simulink model "Back2BackSim1"  (R2017a)
settings: Solver=VariableStepAuto  StartTime=0.0  StopTime=.2  RelTol=1e-3
undefined symbols (not defined in the file or in its folder): st_time3
libraries: fl_lib x62, nesl_utility x32, powerlib_meascontrol x8, powerlib x1, elec_lib x1
(part 1 of 2)
settings Model: Creator=erich  LastModifiedBy=erich

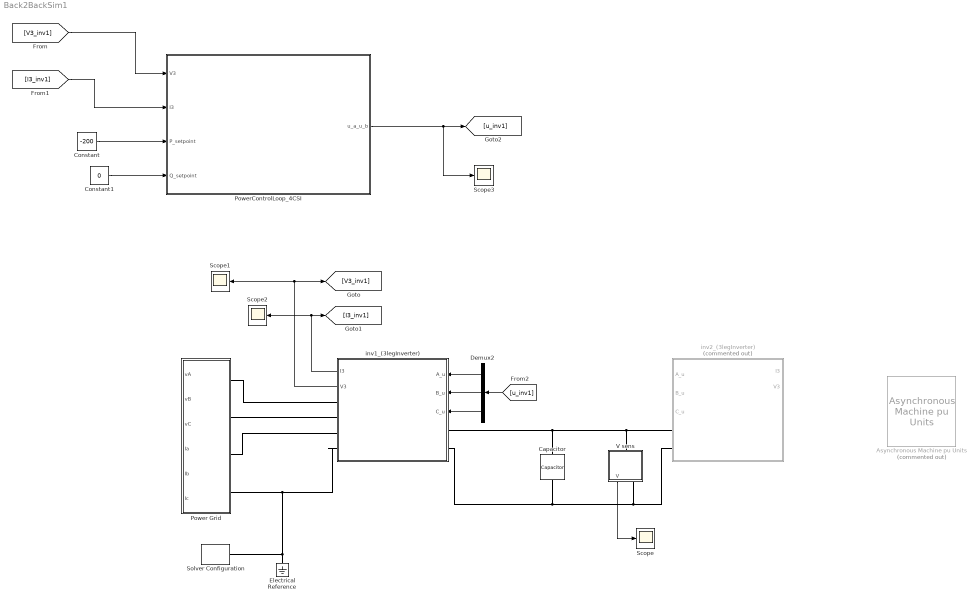
== system Back2BackSim1 ==
  Asynchronous Machine pu Units : powerlib/Machines/Asynchronous Machine pu Units  Commented=on  RotorType=Squirrel-cage  PresetModel=No  MechanicalLoad=Torque Tm  ShowDetailedParameters=on  ReferenceFrame=Rotor  Units=pu  MeasurementBus=off  NominalParameters=[3730 460 60]  Stator=[0.01965 0.0397]  Rotor=[0.01909 0.0397]  Cage1=[0.01909 0.0397]  Cage2=[0.01909 0.0397]  Lm=1.354  Mechanical=[0.09526 0.05479 2]  PolePairs=2  InitialConditions="[ 1,0   0,0,0   0,0,0 ]"  SimulateSaturation=off  Saturation="[0.212,0.4201,0.8125,1.0979,1.4799,2.2457,3.2586,4.5763,6.4763 ;   0.5,0.7,0.9,1,1.1,1.2 ,1.3,1.4,1.5]"  LoadFlowParameters=0  TsPowergui=0  TsBlock=-1  IterativeModel=Trapezoidal non iterative  IterativeDiscreteModel=Trapezoidal non iterative  Pmec=0
      settings: SourceProductName=Simscape Power Systems  SourceProductBaseCode=PS
  Capacitor : elec_lib/Passive Devices/Capacitor  enable_table=0  c=100 uF  Cvec=[1.0e-5, 1.0e-6] F  Vvec=[0.0, 10.0] V  CV_table_symmetry=1  C_tol=5  enable_C_tol=0  tol_distribution=1  nSigma=4  r=1e-6 Ohm  g=0 1/Ohm  enable_operating_limits=0  operating_limit_action=2  max_working_voltage_range=[-25.0, 25.0] V  power_rating=1 W  enable_faults=0  fault_action=1  Cscale_faulted=100  R_faulted=1e-3 Ohm  G_faulted=0 1/Ohm  tau_fault=1e-3 s  enable_temporal_fault=0  t_fault=1 s  enable_behavioral_fault=0  max_permissible_voltage_range=[-100.0, 100.0] V  t_fail_on_voltage=1 s  i_specify=off  i_priority=None  i=0 A  i_nominal_specify=off  i_nominal_unit=A  i_nominal_value=1  v_specify=off  v_priority=None  v=0 V  v_nominal_specify=off  v_nominal_unit=V  v_nominal_value=1  vc_specify=off  vc_priority=High  vc=0 V  vc_nominal_specify=off  vc_nominal_unit=V  vc_nominal_value=1
  Constant : Constant  Value=-200
  Constant1 : Constant  Value=0
  Demux2 : Demux  Outputs=3
  Electrical Reference : fl_lib/Electrical/Electrical Elements/Electrical Reference
  Power Grid : Subsystem
  PowerControlLoop_4CSI : Subsystem
      mask Display:
      | port_label('input', 1, '\fontsize{14} V_{abc}', 'texmode', 'on')
      | port_label('input', 2, '\fontsize{14} I_{abc}', 'texmode', 'on')
      | port_label('input', 3, '\fontsize{14} P_{set}', 'texmode', 'on')
      | port_label('input', 4, '\fontsize{14} Q_{set}', 'texmode', 'on')
      | port_label('output', 1, '\fontsize{14} u_{\alpha, \beta}', 'texmode', 'on')
      | 
      | 
      | disp('\fontsize{12} Power Control for 3\Phi CSI', 'texmode', 'on')
  Scope{,1..3} (4 alike) : Scope
  Solver Configuration : nesl_utility/Solver Configuration  PhysicalDomain=network_engine_domain  SubClassName=solver  LeftPortType=input  RightPortType=generic  Accelerate=off  Tones=[]  Harmonics=[]  SimulateNoise=off  Profile=off  UseLocalSampling=off  EnableSwitchedLinearOptims=on  FrequencyDomain=off  UseCCode=off  RelTol=0.001  AbsTol=1e-06  MinStep=1e-09  ToWorkspace=off  RevertToSquareIcSolve=off  NumHomotopyIterations=100  PhasorMode=off  PhasorModeNumHarmonics=1  OverrideAbsTol=off  DoDC=off  ResidualTolerance=1e-09  UseLocalSolver=on  LocalSolverChoice=NE_BACKWARD_EULER_ADVANCER  LocalSolverSampleTime=1e-6  DoFixedCost=on  MaxNonlinIter=3  MaxModeIter=2  LinearAlgebra=Sparse  DelaysMemoryBudget=1024  AutomaticFiltering=on  FilteringTimeConstant=0.001
  V sens : Subsystem
      mask Display:
      | port_label('lconn', 1, '+')
      | port_label('rconn', 1, '-')
      | port_label('output', 1, 'V')
      | 
      | 
      | x=.5+[-.31:.01:.31];
      | y=sqrt(.1-(x-.5).^2)+.4;
      | y2=-sqrt(.1-(x-.5).^2)+.5;
      | 
      | plot(x, y)
      | plot(x, y2)
      | 
      | text(.47, .5,'V', 'texmode', 'on')
      | 
      | plot([.1 .22], [.44 .44])
      | plot([.8 .9], [.44 .44])
  inv1_(3legInverter) : Subsystem
      mask Display:
      | port_label('input', 1, 'A_u')
      | port_label('input', 2, 'B_u')
      | port_label('input', 3, 'C_u')
      | 
      | port_label('lconn', 1, 'DC +')
      | port_label('lconn', 2, 'DC -')
      | 
      | 
      | port_label('rconn', 1, 'A')
      | port_label('rconn', 2, 'B')
      | port_label('rconn', 3, 'C')
      | 
      | port_label('output', 1, 'I_{3\Phi}', 'texmode', 'on')
      | port_label('output', 2, 'V_{3\Phi}', 'texmode', 'on')
      | 
      | plot([0.1 .9]-.06, [0.1 .9])
      | plot([0.2 .4], [.7 .7])
      | plot([0.2 .24], [.65 .65])
      | plot([0.28 .32], [.65 .65])
      | plot([0.36 .40], [.65 .65])
      | 
      | plot([.5:.01:.7], .25+sin(30*[.2:.01:.4])/10)
  inv2_(3legInverter) : Subsystem  Commented=on
      mask Display:
      | port_label('input', 1, 'A_u')
      | port_label('input', 2, 'B_u')
      | port_label('input', 3, 'C_u')
      | 
      | port_label('lconn', 1, 'DC +')
      | port_label('lconn', 2, 'DC -')
      | 
      | 
      | port_label('rconn', 1, 'A')
      | port_label('rconn', 2, 'B')
      | port_label('rconn', 3, 'C')
      | 
      | port_label('output', 1, 'I_{3\Phi}', 'texmode', 'on')
      | port_label('output', 2, 'V_{3\Phi}', 'texmode', 'on')
      | 
      | plot([0.1 .9]-.06, [0.1 .9])
      | plot([0.2 .4], [.7 .7])
      | plot([0.2 .24], [.65 .65])
      | plot([0.28 .32], [.65 .65])
      | plot([0.36 .40], [.65 .65])
      | 
      | plot([.5:.01:.7], .25+sin(30*[.2:.01:.4])/10)
  wires:
  inv1_(3legInverter)/2(V3) -> [V3_inv1], Scope1/1
  inv1_(3legInverter)/1(I3) -> Scope2/1, [I3_inv1]
  Demux2/3 -> inv1_(3legInverter)/3(C_u)
  Demux2/2 -> inv1_(3legInverter)/2(B_u)
  Demux2/1 -> inv1_(3legInverter)/1(A_u)
  [u_inv1] -> Demux2/1
  V sens/1(V) -> Scope/1
  PowerControlLoop_4CSI/1(u_a_u_b) -> Scope3/1, [u_inv1]
  [V3_inv1] -> PowerControlLoop_4CSI/1(V3)
  [I3_inv1] -> PowerControlLoop_4CSI/2(I3)
  Constant/1 -> PowerControlLoop_4CSI/3(P_setpoint)
  Constant1/1 -> PowerControlLoop_4CSI/4(Q_setpoint)
  connections:
  inv1_(3legInverter)/RConn2 -- Power Grid/LConn2
  inv1_(3legInverter)/RConn3 -- Power Grid/LConn3
  inv1_(3legInverter)/RConn1 -- Power Grid/LConn1
  inv1_(3legInverter)/LConn1 -- V sens/LConn1 -- inv2_(3legInverter)/LConn1 -- Capacitor/LConn1
  Capacitor/RConn1 -- V sens/RConn1 -- inv2_(3legInverter)/LConn2 -- inv1_(3legInverter)/LConn2
  Power Grid/LConn4 -- Solver Configuration/RConn1 -- Electrical Reference/LConn1 -- inv1_(3legInverter)/RConn4

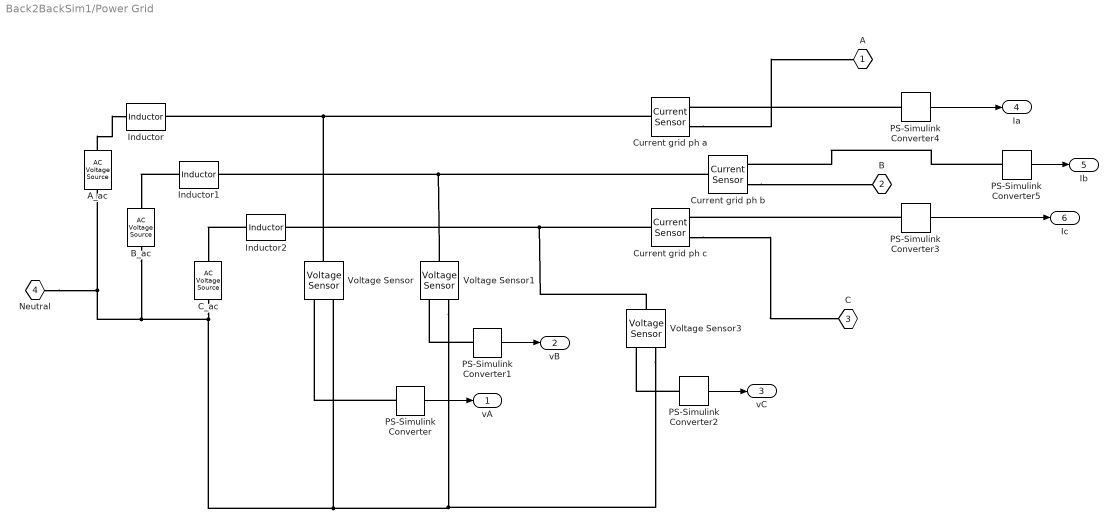
== system Back2BackSim1/Power Grid ==
  A_ac : fl_lib/Electrical/Electrical Sources/AC Voltage Source  amp=170 V  shift=0 deg  frequency=60 Hz  omega=0 rad/s
  B_ac : fl_lib/Electrical/Electrical Sources/AC Voltage Source  amp=170 V  shift=-120 deg  frequency=60 Hz  omega=0 rad/s
  C_ac : fl_lib/Electrical/Electrical Sources/AC Voltage Source  amp=170 V  shift=120 deg  frequency=60 Hz  omega=0 rad/s
  Current grid ph a : fl_lib/Electrical/Electrical Sensors/Current Sensor
  Current grid ph b : fl_lib/Electrical/Electrical Sensors/Current Sensor
  Current grid ph c : fl_lib/Electrical/Electrical Sensors/Current Sensor
  Inductor : fl_lib/Electrical/Electrical Elements/Inductor  l=0.1 uH  r=0.2 Ohm  g=1e-9 1/Ohm  i_specify=off  i_priority=None  i=0 A  i_nominal_specify=off  i_nominal_unit=A  i_nominal_value=1  v_specify=off  v_priority=None  v=0 V  v_nominal_specify=off  v_nominal_unit=V  v_nominal_value=1  i_L_specify=on  i_L_priority=High  i_L=0 A  i_L_nominal_specify=off  i_L_nominal_unit=A  i_L_nominal_value=1
  Inductor1 : fl_lib/Electrical/Electrical Elements/Inductor  l=0.1 uH  r=0.2 Ohm  g=1e-9 1/Ohm  i_specify=off  i_priority=None  i=0 A  i_nominal_specify=off  i_nominal_unit=A  i_nominal_value=1  v_specify=off  v_priority=None  v=0 V  v_nominal_specify=off  v_nominal_unit=V  v_nominal_value=1  i_L_specify=on  i_L_priority=High  i_L=0 A  i_L_nominal_specify=off  i_L_nominal_unit=A  i_L_nominal_value=1
  Inductor2 : fl_lib/Electrical/Electrical Elements/Inductor  l=0.1 uH  r=0.2 Ohm  g=1e-9 1/Ohm  i_specify=off  i_priority=None  i=0 A  i_nominal_specify=off  i_nominal_unit=A  i_nominal_value=1  v_specify=off  v_priority=None  v=0 V  v_nominal_specify=off  v_nominal_unit=V  v_nominal_value=1  i_L_specify=on  i_L_priority=High  i_L=0 A  i_L_nominal_specify=off  i_L_nominal_unit=A  i_L_nominal_value=1
  PS-Simulink Converter{,1..5} (6 alike) : nesl_utility/PS-Simulink Converter  PhysicalDomain=network_engine_domain  SubClassName=ps_output  LeftPortType=input  RightPortType=output  PseudoPeriodic=off  Frequencies=[]  Unit=1  AffineConversion=off
  Voltage Sensor : fl_lib/Electrical/Electrical Sensors/Voltage Sensor
  Voltage Sensor1 : fl_lib/Electrical/Electrical Sensors/Voltage Sensor
  Voltage Sensor3 : fl_lib/Electrical/Electrical Sensors/Voltage Sensor
  A : PMIOPort  Port=1  Side=Left
  B : PMIOPort  Port=2  Side=Left
  C : PMIOPort  Port=3  Side=Left
  Neutral : PMIOPort  Port=4  Side=Left
  vA : Outport
  vB : Outport  Port=2
  vC : Outport  Port=3
  Ia : Outport  Port=4
  Ib : Outport  Port=5
  Ic : Outport  Port=6
  wires:
  PS-Simulink Converter/1 -> vA/1
  PS-Simulink Converter1/1 -> vB/1
  PS-Simulink Converter2/1 -> vC/1
  PS-Simulink Converter4/1 -> Ia/1
  PS-Simulink Converter5/1 -> Ib/1
  PS-Simulink Converter3/1 -> Ic/1
  connections:
  Inductor2/LConn1 -- C_ac/LConn1
  A_ac/LConn1 -- Inductor/LConn1
  Inductor1/LConn1 -- B_ac/LConn1
  Voltage Sensor1/LConn1 -- Inductor1/RConn1 -- Current grid ph b/LConn1
  PS-Simulink Converter/LConn1 -- Voltage Sensor/RConn1
  Voltage Sensor3/LConn1 -- Inductor2/RConn1 -- Current grid ph c/LConn1
  Voltage Sensor/LConn1 -- Current grid ph a/LConn1 -- Inductor/RConn1
  A_ac/RConn1 -- Neutral/RConn1 -- Voltage Sensor3/RConn2 -- Voltage Sensor1/RConn2 -- Voltage Sensor/RConn2 -- C_ac/RConn1 -- B_ac/RConn1
  PS-Simulink Converter1/LConn1 -- Voltage Sensor1/RConn1
  PS-Simulink Converter2/LConn1 -- Voltage Sensor3/RConn1
  Current grid ph c/RConn2 -- C/RConn1
  Current grid ph b/RConn2 -- B/RConn1
  Current grid ph a/RConn2 -- A/RConn1
  PS-Simulink Converter3/LConn1 -- Current grid ph c/RConn1
  PS-Simulink Converter4/LConn1 -- Current grid ph a/RConn1
  PS-Simulink Converter5/LConn1 -- Current grid ph b/RConn1

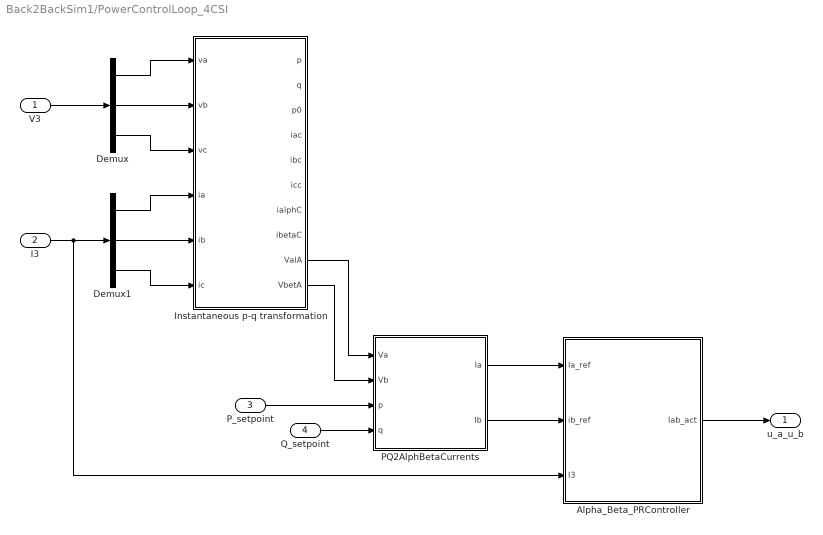
== system Back2BackSim1/PowerControlLoop_4CSI ==
  V3 : Inport
  I3 : Inport  Port=2
  P_setpoint : Inport  Port=3
  Q_setpoint : Inport  Port=4
  Alpha_Beta_PRController : Subsystem
      mask Display:
      | port_label('input', 1, '\fontsize{13} \alpha_{ref}', 'texmode', 'on')
      | port_label('input', 2, '\fontsize{13} \beta_{ref}', 'texmode', 'on')
      | port_label('input', 3, '\fontsize{13} [ a, b, c ]', 'texmode', 'on')
      | 
      | port_label('output', 1, '\fontsize{13} [ u_{a}, u_{b}, u_{c} ]', 'texmode', 'on')
      | 
      | 
      | %plot([.4 .6],.05+[.5 .7])
      | %plot([.4 .6],.05+[.9 .7])
      | %plot([.4 .4],.05+[.9 .5])
      | 
      | text(.53,.2,'\fontsize{25} \int', 'texmode', 'on')
      | plot(.65+[0:.01:pi/10], .2+sin(40*[0:.01:pi/10])/13)
      | 
      | %text(.5,.8,'\fontsize{15} PR_{\alpha \beta}', 'texmode', 'on')
  Demux : Demux  Outputs=3
  Demux1 : Demux  Outputs=3
  Instantaneous p-q transformation : MATLAB Function  TreatAsAtomicUnit=on
  PQ2AlphBetaCurrents : MATLAB Function  TreatAsAtomicUnit=on
  u_a_u_b : Outport
  wires:
  I3/1 -> Alpha_Beta_PRController/3(I3), Demux1/1
  PQ2AlphBetaCurrents/1(Ia) -> Alpha_Beta_PRController/1(Ia_ref)
  V3/1 -> Demux/1
  Alpha_Beta_PRController/1(Iab_act) -> u_a_u_b/1
  Demux/1 -> Instantaneous p-q transformation/1(va)
  Demux1/3 -> Instantaneous p-q transformation/6(ic)
  Demux1/1 -> Instantaneous p-q transformation/4(ia)
  Demux1/2 -> Instantaneous p-q transformation/5(ib)
  P_setpoint/1 -> PQ2AlphBetaCurrents/3(p)
  Q_setpoint/1 -> PQ2AlphBetaCurrents/4(q)
  PQ2AlphBetaCurrents/2(Ib) -> Alpha_Beta_PRController/2(ib_ref)
  Demux/3 -> Instantaneous p-q transformation/3(vc)
  Instantaneous p-q transformation/9(ValA) -> PQ2AlphBetaCurrents/1(Va)
  Instantaneous p-q transformation/10(VbetA) -> PQ2AlphBetaCurrents/2(Vb)
  Demux/2 -> Instantaneous p-q transformation/2(vb)

== system Back2BackSim1/V sens ==
  PS-Simulink Converter : nesl_utility/PS-Simulink Converter  PhysicalDomain=network_engine_domain  SubClassName=ps_output  LeftPortType=input  RightPortType=output  PseudoPeriodic=off  Frequencies=[]  Unit=1  AffineConversion=off
  Voltage Sensor : fl_lib/Electrical/Electrical Sensors/Voltage Sensor
  + : PMIOPort  Port=1  Side=Left
  - : PMIOPort  Port=2  Side=Right
  V : Outport
  wires:
  PS-Simulink Converter/1 -> V/1
  connections:
  PS-Simulink Converter/LConn1 -- Voltage Sensor/RConn1
  Voltage Sensor/RConn2 -- -/RConn1
  Voltage Sensor/LConn1 -- +/RConn1

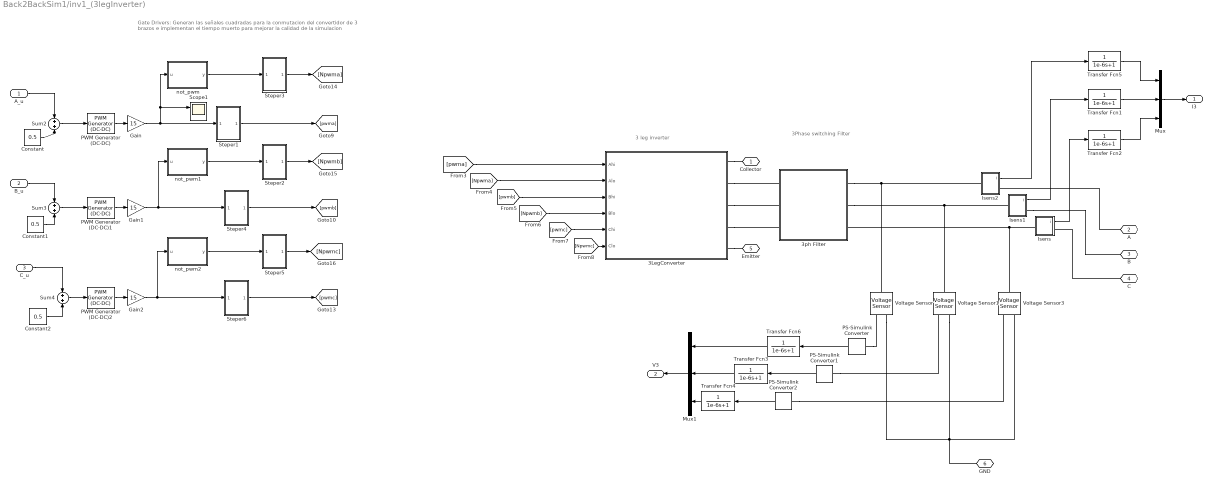
== system Back2BackSim1/inv1_(3legInverter) ==
  note: Gate Drivers: Generan las señales cuadradas para
      | la conmutacion del convertidor de 3 brazos e implementan el
      | tiempo muerto para mejorar la calidad de la simulacion
  note: 3 leg inverter
  note: 3Phase
      | switching
      | Filter
  A_u : Inport
  B_u : Inport  Port=2
  C_u : Inport  Port=3
  3LegConverter : Subsystem
      mask Display:
      | % entradas de conmutacion del mosfet
      | port_label('input',1,'Ahi')
      | port_label('input',2,'Alo')
      | port_label('input',3,'Bhi')
      | port_label('input',4,'Blo')
      | port_label('input',5,'Chi')
      | port_label('input',6,'Clo')
      | 
      | % puertos de conexion del inversor
      | port_label('rconn',1,'Collector') % + fuente dc
      | port_label('rconn',2,'A') % fase A
      | port_label('rconn',3,'B') % fase B
      | port_label('rconn',4,'C') % fase C
      | port_label('rconn',5,'Emitter') % ref fuente dc
      | 
      | 
      | plot([.4 .4],[.35 .7])
      | plot([.2 .4],[.52 .52])
      | plot([.46 .46],[.22 .85])
      | plot([.46 .7],[.73 .73])
      | plot([.46 .7],[.32 .32])
  3ph Filter : Subsystem
  Constant : Constant  Value=0.5
  Constant1 : Constant  Value=0.5
  Constant2 : Constant  Value=0.5
  Gain : Gain  Gain=15
  Gain1 : Gain  Gain=15
  Gain2 : Gain  Gain=15
  Isens : Subsystem
  Isens1 : Subsystem
  Isens2 : Subsystem
  Mux : Mux  Inputs=3
  Mux1 : Mux  Inputs=3
  PS-Simulink Converter : nesl_utility/PS-Simulink Converter  PhysicalDomain=network_engine_domain  SubClassName=ps_output  LeftPortType=input  RightPortType=output  PseudoPeriodic=off  Frequencies=[]  Unit=1  AffineConversion=off
  PS-Simulink Converter1 : nesl_utility/PS-Simulink Converter  PhysicalDomain=network_engine_domain  SubClassName=ps_output  LeftPortType=input  RightPortType=output  PseudoPeriodic=off  Frequencies=[]  Unit=1  AffineConversion=off
  PS-Simulink Converter2 : nesl_utility/PS-Simulink Converter  PhysicalDomain=network_engine_domain  SubClassName=ps_output  LeftPortType=input  RightPortType=output  PseudoPeriodic=off  Frequencies=[]  Unit=1  AffineConversion=off
  PWM Generator (DC-DC) : powerlib_meascontrol/Pulse & Signal Generators/PWM Generator (DC-DC)  Fsw=5000  Ts=0
  PWM Generator (DC-DC)1 : powerlib_meascontrol/Pulse & Signal Generators/PWM Generator (DC-DC)  Fsw=5000  Ts=0
  PWM Generator (DC-DC)2 : powerlib_meascontrol/Pulse & Signal Generators/PWM Generator (DC-DC)  Fsw=5000  Ts=0
  Scope1 : Scope  NumInputPorts=2
  Steper1 : Subsystem
  Steper2 : Subsystem
  Steper3 : Subsystem
  Steper4 : Subsystem
  Steper5 : Subsystem
  Steper6 : Subsystem
  Sum2 : Sum
  Sum3 : Sum
  Sum4 : Sum
  Transfer Fcn{1..6} (6 alike) : TransferFcn  Denominator=[1e-6 1]
  Voltage Sensor : fl_lib/Electrical/Electrical Sensors/Voltage Sensor
  Voltage Sensor1 : fl_lib/Electrical/Electrical Sensors/Voltage Sensor
  Voltage Sensor3 : fl_lib/Electrical/Electrical Sensors/Voltage Sensor
  not_pwm : MATLAB Function  TreatAsAtomicUnit=on
  not_pwm1 : MATLAB Function  TreatAsAtomicUnit=on
  not_pwm2 : MATLAB Function  TreatAsAtomicUnit=on
  Collector : PMIOPort  Port=1  Side=Left
  A : PMIOPort  Port=2  Side=Right
  B : PMIOPort  Port=3  Side=Right
  C : PMIOPort  Port=4  Side=Right
  Emitter : PMIOPort  Port=5  Side=Left
  GND : PMIOPort  Port=6  Side=Right
  I3 : Outport
  V3 : Outport  Port=2
  wires:
  C_u/1 -> Sum4/1
  [Npwmc] -> 3LegConverter/6(Clo)
  [pwma] -> 3LegConverter/1(Ahi)
  [pwmc] -> 3LegConverter/5(Chi)
  [Npwma] -> 3LegConverter/2(Alo)
  [Npwmb] -> 3LegConverter/4(Blo)
  [pwmb] -> 3LegConverter/3(Bhi)
  Steper5/1(Out1) -> [Npwmc]
  Steper4/1(Out1) -> [pwmb]
  Gain/1 -> Steper1/1(In1), Scope1/1, not_pwm/1(u)
  not_pwm1/1(y) -> Steper2/1(In1)
  Steper3/1(Out1) -> [Npwma]
  Constant/1 -> Sum2/2
  Sum2/1 -> PWM Generator (DC-DC)/1
  Gain2/1 -> Steper6/1(In1), not_pwm2/1(u)
  Sum3/1 -> PWM Generator (DC-DC)1/1
  Steper6/1(Out1) -> [pwmc]
  Sum4/1 -> PWM Generator (DC-DC)2/1
  Gain1/1 -> Steper4/1(In1), not_pwm1/1(u)
  not_pwm2/1(y) -> Steper5/1(In1)
  Steper2/1(Out1) -> [Npwmb]
  Constant2/1 -> Sum4/2
  PWM Generator (DC-DC)1/1 -> Gain1/1
  not_pwm/1(y) -> Steper3/1(In1)
  PWM Generator (DC-DC)/1 -> Gain/1
  PWM Generator (DC-DC)2/1 -> Gain2/1
  Steper1/1(Out1) -> [pwma]
  Constant1/1 -> Sum3/2
  B_u/1 -> Sum3/1
  A_u/1 -> Sum2/1
  Isens/1(i) -> Transfer Fcn2/1
  Isens1/1(i) -> Transfer Fcn1/1
  Isens2/1(i) -> Transfer Fcn5/1
  Mux/1 -> I3/1
  Transfer Fcn1/1 -> Mux/2
  Transfer Fcn5/1 -> Mux/1
  Transfer Fcn2/1 -> Mux/3
  Mux1/1 -> V3/1
  PS-Simulink Converter/1 -> Transfer Fcn6/1
  PS-Simulink Converter1/1 -> Transfer Fcn3/1
  PS-Simulink Converter2/1 -> Transfer Fcn4/1
  Transfer Fcn6/1 -> Mux1/1
  Transfer Fcn3/1 -> Mux1/2
  Transfer Fcn4/1 -> Mux1/3
  connections:
  3LegConverter/RConn5 -- Emitter/RConn1
  3LegConverter/RConn1 -- Collector/RConn1
  C/RConn1 -- Isens/RConn1
  Isens1/RConn1 -- B/RConn1
  A/RConn1 -- Isens2/RConn1
  3LegConverter/RConn2 -- 3ph Filter/LConn1
  3LegConverter/RConn3 -- 3ph Filter/LConn2
  3LegConverter/RConn4 -- 3ph Filter/LConn3
  3ph Filter/RConn1 -- Voltage Sensor/LConn1 -- Isens2/LConn1
  3ph Filter/RConn2 -- Isens1/LConn1 -- Voltage Sensor1/LConn1
  Isens/LConn1 -- Voltage Sensor3/LConn1 -- 3ph Filter/RConn3
  Voltage Sensor1/RConn2 -- Voltage Sensor3/RConn2 -- GND/RConn1 -- Voltage Sensor/RConn2
  PS-Simulink Converter1/LConn1 -- Voltage Sensor1/RConn1
  PS-Simulink Converter2/LConn1 -- Voltage Sensor3/RConn1
  PS-Simulink Converter/LConn1 -- Voltage Sensor/RConn1

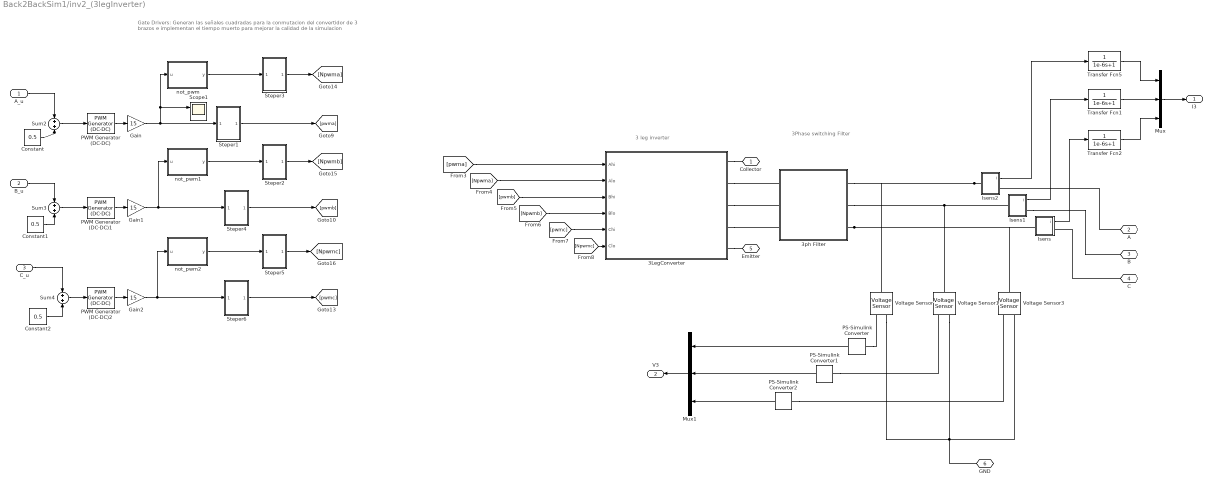
== system Back2BackSim1/inv2_(3legInverter) ==
  note: 3Phase
      | switching
      | Filter
  note: 3 leg inverter
  note: Gate Drivers: Generan las señales cuadradas para
      | la conmutacion del convertidor de 3 brazos e implementan el
      | tiempo muerto para mejorar la calidad de la simulacion
  A_u : Inport
  B_u : Inport  Port=2
  C_u : Inport  Port=3
  3LegConverter : Subsystem
      mask Display:
      | % entradas de conmutacion del mosfet
      | port_label('input',1,'Ahi')
      | port_label('input',2,'Alo')
      | port_label('input',3,'Bhi')
      | port_label('input',4,'Blo')
      | port_label('input',5,'Chi')
      | port_label('input',6,'Clo')
      | 
      | % puertos de conexion del inversor
      | port_label('rconn',1,'Collector') % + fuente dc
      | port_label('rconn',2,'A') % fase A
      | port_label('rconn',3,'B') % fase B
      | port_label('rconn',4,'C') % fase C
      | port_label('rconn',5,'Emitter') % ref fuente dc
      | 
      | 
      | plot([.4 .4],[.35 .7])
      | plot([.2 .4],[.52 .52])
      | plot([.46 .46],[.22 .85])
      | plot([.46 .7],[.73 .73])
      | plot([.46 .7],[.32 .32])
  3ph Filter : Subsystem
  Constant : Constant  Value=0.5
  Constant1 : Constant  Value=0.5
  Constant2 : Constant  Value=0.5
  Gain : Gain  Gain=15
  Gain1 : Gain  Gain=15
  Gain2 : Gain  Gain=15
  Isens : Subsystem
  Isens1 : Subsystem
  Isens2 : Subsystem
  Mux : Mux  Inputs=3
  Mux1 : Mux  Inputs=3
  PS-Simulink Converter : nesl_utility/PS-Simulink Converter  PhysicalDomain=network_engine_domain  SubClassName=ps_output  LeftPortType=input  RightPortType=output  PseudoPeriodic=off  Frequencies=[]  Unit=1  AffineConversion=off
  PS-Simulink Converter1 : nesl_utility/PS-Simulink Converter  PhysicalDomain=network_engine_domain  SubClassName=ps_output  LeftPortType=input  RightPortType=output  PseudoPeriodic=off  Frequencies=[]  Unit=1  AffineConversion=off
  PS-Simulink Converter2 : nesl_utility/PS-Simulink Converter  PhysicalDomain=network_engine_domain  SubClassName=ps_output  LeftPortType=input  RightPortType=output  PseudoPeriodic=off  Frequencies=[]  Unit=1  AffineConversion=off
  PWM Generator (DC-DC) : powerlib_meascontrol/Pulse & Signal Generators/PWM Generator (DC-DC)  Fsw=5000  Ts=0
  PWM Generator (DC-DC)1 : powerlib_meascontrol/Pulse & Signal Generators/PWM Generator (DC-DC)  Fsw=5000  Ts=0
  PWM Generator (DC-DC)2 : powerlib_meascontrol/Pulse & Signal Generators/PWM Generator (DC-DC)  Fsw=5000  Ts=0
  Scope1 : Scope  NumInputPorts=2
  Steper1 : Subsystem
  Steper2 : Subsystem
  Steper3 : Subsystem
  Steper4 : Subsystem
  Steper5 : Subsystem
  Steper6 : Subsystem
  Sum2 : Sum
  Sum3 : Sum
  Sum4 : Sum
  Transfer Fcn1 : TransferFcn  Denominator=[1e-6 1]
  Transfer Fcn2 : TransferFcn  Denominator=[1e-6 1]
  Transfer Fcn5 : TransferFcn  Denominator=[1e-6 1]
  Voltage Sensor : fl_lib/Electrical/Electrical Sensors/Voltage Sensor
  Voltage Sensor1 : fl_lib/Electrical/Electrical Sensors/Voltage Sensor
  Voltage Sensor3 : fl_lib/Electrical/Electrical Sensors/Voltage Sensor
  not_pwm : MATLAB Function  TreatAsAtomicUnit=on
  not_pwm1 : MATLAB Function  TreatAsAtomicUnit=on
  not_pwm2 : MATLAB Function  TreatAsAtomicUnit=on
  Collector : PMIOPort  Port=1  Side=Left
  A : PMIOPort  Port=2  Side=Right
  B : PMIOPort  Port=3  Side=Right
  C : PMIOPort  Port=4  Side=Right
  Emitter : PMIOPort  Port=5  Side=Left
  GND : PMIOPort  Port=6  Side=Right
  I3 : Outport
  V3 : Outport  Port=2
  wires:
  PS-Simulink Converter2/1 -> Mux1/3
  PS-Simulink Converter1/1 -> Mux1/2
  PS-Simulink Converter/1 -> Mux1/1
  Mux1/1 -> V3/1
  Transfer Fcn2/1 -> Mux/3
  Transfer Fcn5/1 -> Mux/1
  Transfer Fcn1/1 -> Mux/2
  Mux/1 -> I3/1
  Isens2/1(i) -> Transfer Fcn5/1
  Isens1/1(i) -> Transfer Fcn1/1
  Isens/1(i) -> Transfer Fcn2/1
  A_u/1 -> Sum2/1
  B_u/1 -> Sum3/1
  Constant1/1 -> Sum3/2
  Steper1/1(Out1) -> [pwma]
  PWM Generator (DC-DC)2/1 -> Gain2/1
  PWM Generator (DC-DC)/1 -> Gain/1
  not_pwm/1(y) -> Steper3/1(In1)
  PWM Generator (DC-DC)1/1 -> Gain1/1
  Constant2/1 -> Sum4/2
  Steper2/1(Out1) -> [Npwmb]
  not_pwm2/1(y) -> Steper5/1(In1)
  Gain1/1 -> not_pwm1/1(u), Steper4/1(In1)
  Sum4/1 -> PWM Generator (DC-DC)2/1
  Steper6/1(Out1) -> [pwmc]
  Sum3/1 -> PWM Generator (DC-DC)1/1
  Gain2/1 -> not_pwm2/1(u), Steper6/1(In1)
  Sum2/1 -> PWM Generator (DC-DC)/1
  Constant/1 -> Sum2/2
  Steper3/1(Out1) -> [Npwma]
  not_pwm1/1(y) -> Steper2/1(In1)
  Gain/1 -> not_pwm/1(u), Scope1/1, Steper1/1(In1)
  Steper4/1(Out1) -> [pwmb]
  Steper5/1(Out1) -> [Npwmc]
  [pwmb] -> 3LegConverter/3(Bhi)
  [Npwmb] -> 3LegConverter/4(Blo)
  [Npwma] -> 3LegConverter/2(Alo)
  [pwmc] -> 3LegConverter/5(Chi)
  [pwma] -> 3LegConverter/1(Ahi)
  [Npwmc] -> 3LegConverter/6(Clo)
  C_u/1 -> Sum4/1
  connections:
  PS-Simulink Converter/LConn1 -- Voltage Sensor/RConn1
  PS-Simulink Converter2/LConn1 -- Voltage Sensor3/RConn1
  PS-Simulink Converter1/LConn1 -- Voltage Sensor1/RConn1
  Voltage Sensor/RConn2 -- GND/RConn1 -- Voltage Sensor3/RConn2 -- Voltage Sensor1/RConn2
  3ph Filter/RConn3 -- Voltage Sensor3/LConn1 -- Isens/LConn1
  Voltage Sensor1/LConn1 -- Isens1/LConn1 -- 3ph Filter/RConn2
  Isens2/LConn1 -- Voltage Sensor/LConn1 -- 3ph Filter/RConn1
  3LegConverter/RConn4 -- 3ph Filter/LConn3
  3LegConverter/RConn3 -- 3ph Filter/LConn2
  3LegConverter/RConn2 -- 3ph Filter/LConn1
  A/RConn1 -- Isens2/RConn1
  Isens1/RConn1 -- B/RConn1
  C/RConn1 -- Isens/RConn1
  3LegConverter/RConn1 -- Collector/RConn1
  3LegConverter/RConn5 -- Emitter/RConn1

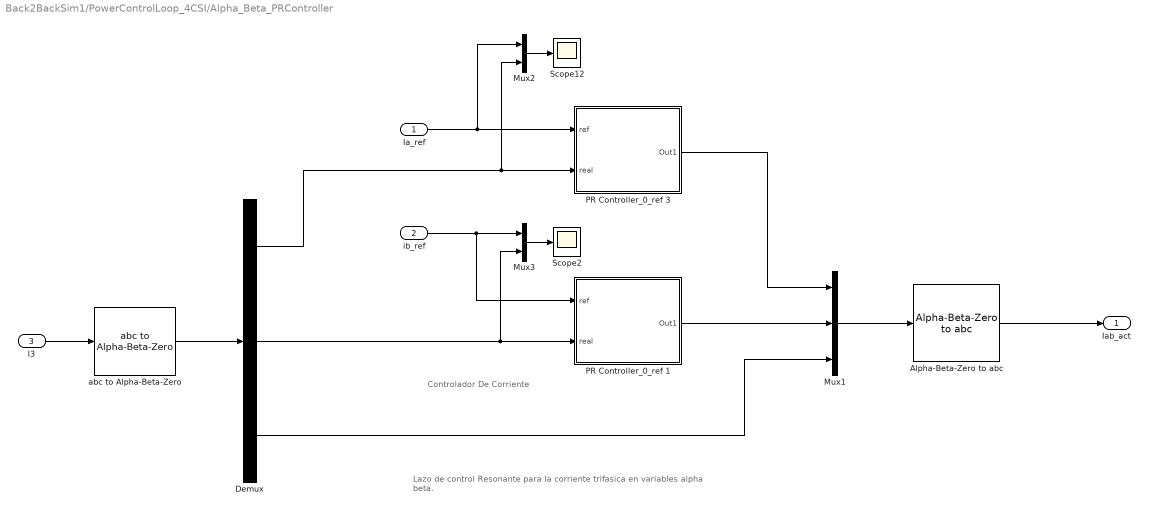
== system Back2BackSim1/PowerControlLoop_4CSI/Alpha_Beta_PRController ==
  note: Controlador De Corriente
  note: Lazo de control Resonante para la
      | corriente trifasica en variables alpha beta.
  Ia_ref : Inport
  ib_ref : Inport  Port=2
  I3 : Inport  Port=3
  Alpha-Beta-Zero to abc : powerlib_meascontrol/Transformations/Alpha-Beta-Zero to abc
      settings: SourceProductName=Simscape Power Systems  SourceProductBaseCode=PS
  Demux : Demux  Outputs=3
  Mux1 : Mux  Inputs=3
  Mux2 : Mux  Inputs=2
  Mux3 : Mux  Inputs=2
  PR Controller_0_ref 1 : Subsystem
      mask Display:
      | port_label('input',1,'ref')
      | port_label('input',2,'sens')
      | port_label('output',1,'out')
      | 
      | plot(.4+[0:.01:pi/10], .32+sin(40*[0:.01:pi/10])/13)
      | 
      | plot([.4 .6],.05+[.5 .7])
      | plot([.4 .6],.05+[.9 .7])
      | plot([.4 .4],.05+[.9 .5])
      | 
      | text(.27,.37,'\fontsize{25} \int', 'texmode', 'on')
  PR Controller_0_ref 3 : Subsystem
      mask Display:
      | port_label('input',1,'ref')
      | port_label('input',2,'sens')
      | port_label('output',1,'out')
      | 
      | plot(.4+[0:.01:pi/10], .32+sin(40*[0:.01:pi/10])/13)
      | 
      | plot([.4 .6],.05+[.5 .7])
      | plot([.4 .6],.05+[.9 .7])
      | plot([.4 .4],.05+[.9 .5])
      | 
      | text(.27,.37,'\fontsize{25} \int', 'texmode', 'on')
  Scope12 : Scope
  Scope2 : Scope
  abc to Alpha-Beta-Zero : powerlib_meascontrol/Transformations/abc to Alpha-Beta-Zero
      settings: SourceProductName=Simscape Power Systems
  Iab_act : Outport
  wires:
  I3/1 -> abc to Alpha-Beta-Zero/1
  Mux2/1 -> Scope12/1
  Demux/2 -> PR Controller_0_ref 1/2(real), Mux3/2
  PR Controller_0_ref 1/1(Out1) -> Mux1/2
  Mux1/1 -> Alpha-Beta-Zero to abc/1
  Mux3/1 -> Scope2/1
  Alpha-Beta-Zero to abc/1 -> Iab_act/1
  abc to Alpha-Beta-Zero/1 -> Demux/1
  ib_ref/1 -> PR Controller_0_ref 1/1(ref), Mux3/1
  Ia_ref/1 -> Mux2/1, PR Controller_0_ref 3/1(ref)
  PR Controller_0_ref 3/1(Out1) -> Mux1/1
  Demux/3 -> Mux1/3
  Demux/1 -> Mux2/2, PR Controller_0_ref 3/2(real)

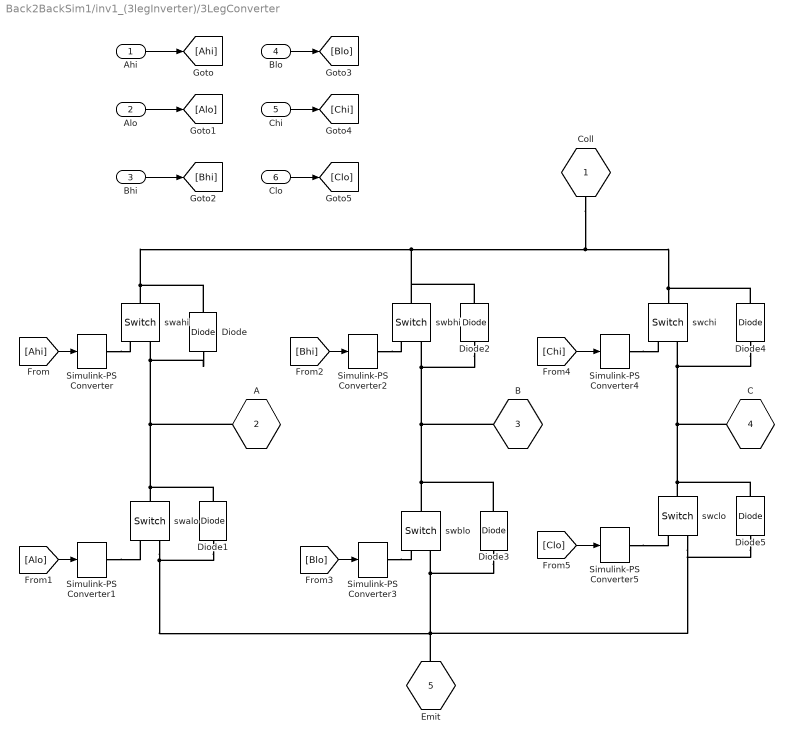
== system Back2BackSim1/inv1_(3legInverter)/3LegConverter ==
  Ahi : Inport
  Alo : Inport  Port=2
  Bhi : Inport  Port=3
  Blo : Inport  Port=4
  Chi : Inport  Port=5
  Clo : Inport  Port=6
  Diode{,1..5} (6 alike) : fl_lib/Electrical/Electrical Elements/Diode  Vf=0.6 V  Ron=0.3 Ohm  Goff=1e-8 1/Ohm  i_specify=off  i_priority=None  i=0 A  i_nominal_specify=off  i_nominal_unit=A  i_nominal_value=1  v_specify=off  v_priority=None  v=0 V  v_nominal_specify=off  v_nominal_unit=V  v_nominal_value=1
  Simulink-PS Converter{,1..5} (6 alike) : nesl_utility/Simulink-PS Converter  PhysicalDomain=network_engine_domain  SubClassName=ps_input  LeftPortType=input  RightPortType=output  PseudoPeriodic=off  Frequencies=[]  NoiseDistribution=none  NoiseParameters=[]  Unit=1  AffineConversion=off  FilteringAndDerivatives=zero  SimscapeFilterOrder=1  InputFilterTimeConstant=0.001  UdotUserProvided=1
  swahi : fl_lib/Electrical/Electrical Elements/Switch  R_closed=0.01 Ohm  G_open=1e-8 1/Ohm  Threshold=2  i_specify=off  i_priority=None  i=0 A  i_nominal_specify=off  i_nominal_unit=A  i_nominal_value=1  v_specify=off  v_priority=None  v=0 V  v_nominal_specify=off  v_nominal_unit=V  v_nominal_value=1
      settings: SourceProductName=Simscape
  swalo : fl_lib/Electrical/Electrical Elements/Switch  R_closed=0.01 Ohm  G_open=1e-8 1/Ohm  Threshold=2  i_specify=off  i_priority=None  i=0 A  i_nominal_specify=off  i_nominal_unit=A  i_nominal_value=1  v_specify=off  v_priority=None  v=0 V  v_nominal_specify=off  v_nominal_unit=V  v_nominal_value=1
      settings: SourceProductName=Simscape
  swbhi : fl_lib/Electrical/Electrical Elements/Switch  R_closed=0.01 Ohm  G_open=1e-8 1/Ohm  Threshold=2  i_specify=off  i_priority=None  i=0 A  i_nominal_specify=off  i_nominal_unit=A  i_nominal_value=1  v_specify=off  v_priority=None  v=0 V  v_nominal_specify=off  v_nominal_unit=V  v_nominal_value=1
      settings: SourceProductName=Simscape
  swblo : fl_lib/Electrical/Electrical Elements/Switch  R_closed=0.01 Ohm  G_open=1e-8 1/Ohm  Threshold=2  i_specify=off  i_priority=None  i=0 A  i_nominal_specify=off  i_nominal_unit=A  i_nominal_value=1  v_specify=off  v_priority=None  v=0 V  v_nominal_specify=off  v_nominal_unit=V  v_nominal_value=1
      settings: SourceProductName=Simscape
  swchi : fl_lib/Electrical/Electrical Elements/Switch  R_closed=0.01 Ohm  G_open=1e-8 1/Ohm  Threshold=2  i_specify=off  i_priority=None  i=0 A  i_nominal_specify=off  i_nominal_unit=A  i_nominal_value=1  v_specify=off  v_priority=None  v=0 V  v_nominal_specify=off  v_nominal_unit=V  v_nominal_value=1
      settings: SourceProductName=Simscape
  swclo : fl_lib/Electrical/Electrical Elements/Switch  R_closed=0.01 Ohm  G_open=1e-8 1/Ohm  Threshold=2  i_specify=off  i_priority=None  i=0 A  i_nominal_specify=off  i_nominal_unit=A  i_nominal_value=1  v_specify=off  v_priority=None  v=0 V  v_nominal_specify=off  v_nominal_unit=V  v_nominal_value=1
      settings: SourceProductName=Simscape
  Coll : PMIOPort  Port=1  Side=Right
  A : PMIOPort  Port=2  Side=Right
  B : PMIOPort  Port=3  Side=Right
  C : PMIOPort  Port=4  Side=Right
  Emit : PMIOPort  Port=5  Side=Right
  wires:
  [Alo] -> Simulink-PS Converter1/1
  [Ahi] -> Simulink-PS Converter/1
  Clo/1 -> [Clo]
  Alo/1 -> [Alo]
  [Blo] -> Simulink-PS Converter3/1
  [Clo] -> Simulink-PS Converter5/1
  Bhi/1 -> [Bhi]
  [Bhi] -> Simulink-PS Converter2/1
  Ahi/1 -> [Ahi]
  [Chi] -> Simulink-PS Converter4/1
  Blo/1 -> [Blo]
  Chi/1 -> [Chi]
  connections:
  swalo/RConn2 -- Diode3/LConn1 -- swblo/RConn2 -- Emit/RConn1 -- Diode5/LConn1 -- swclo/RConn2 -- Diode1/LConn1
  Simulink-PS Converter4/RConn1 -- swchi/RConn1
  Simulink-PS Converter5/RConn1 -- swclo/RConn1
  Simulink-PS Converter/RConn1 -- swahi/RConn1
  swblo/LConn1 -- Diode3/RConn1 -- B/RConn1 -- Diode2/LConn1 -- swbhi/RConn2
  Simulink-PS Converter3/RConn1 -- swblo/RConn1
  Simulink-PS Converter2/RConn1 -- swbhi/RConn1
  Simulink-PS Converter1/RConn1 -- swalo/RConn1
  swalo/LConn1 -- A/RConn1 -- Diode/LConn1 -- swahi/RConn2 -- Diode1/RConn1
  swahi/LConn1 -- Diode/RConn1 -- Diode2/RConn1 -- swbhi/LConn1 -- Coll/RConn1 -- Diode4/RConn1 -- swchi/LConn1
  swclo/LConn1 -- Diode5/RConn1 -- C/RConn1 -- Diode4/LConn1 -- swchi/RConn2

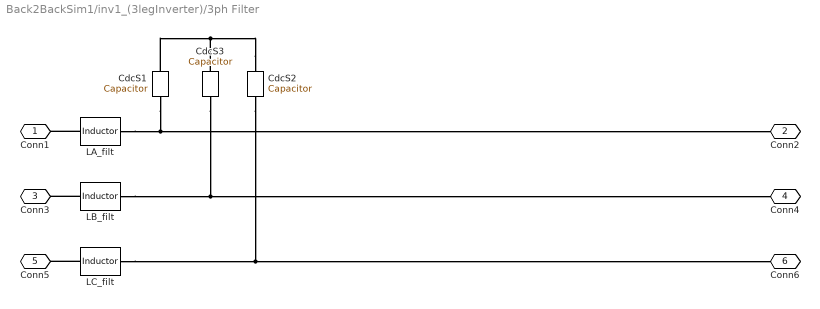
== system Back2BackSim1/inv1_(3legInverter)/3ph Filter ==
  CdcS1 : fl_lib/Electrical/Electrical Elements/Capacitor  c=3.5 uF  r=1e-6 Ohm  g=0 1/Ohm  i_specify=off  i_priority=None  i=0 A  i_nominal_specify=off  i_nominal_unit=A  i_nominal_value=1  v_specify=off  v_priority=None  v=0 V  v_nominal_specify=off  v_nominal_unit=V  v_nominal_value=1  vc_specify=on  vc_priority=High  vc=0 V  vc_nominal_specify=off  vc_nominal_unit=V  vc_nominal_value=1
  CdcS2 : fl_lib/Electrical/Electrical Elements/Capacitor  c=3.5 uF  r=1e-6 Ohm  g=0 1/Ohm  i_specify=off  i_priority=None  i=0 A  i_nominal_specify=off  i_nominal_unit=A  i_nominal_value=1  v_specify=off  v_priority=None  v=0 V  v_nominal_specify=off  v_nominal_unit=V  v_nominal_value=1  vc_specify=on  vc_priority=High  vc=0 V  vc_nominal_specify=off  vc_nominal_unit=V  vc_nominal_value=1
  CdcS3 : fl_lib/Electrical/Electrical Elements/Capacitor  c=3.5 uF  r=1e-6 Ohm  g=0 1/Ohm  i_specify=off  i_priority=None  i=0 A  i_nominal_specify=off  i_nominal_unit=A  i_nominal_value=1  v_specify=off  v_priority=None  v=0 V  v_nominal_specify=off  v_nominal_unit=V  v_nominal_value=1  vc_specify=on  vc_priority=High  vc=0 V  vc_nominal_specify=off  vc_nominal_unit=V  vc_nominal_value=1
  LA_filt : fl_lib/Electrical/Electrical Elements/Inductor  l=6.2 mH  r=0.1 Ohm  g=1e-6 1/Ohm  i_specify=off  i_priority=None  i=0 A  i_nominal_specify=off  i_nominal_unit=A  i_nominal_value=1  v_specify=off  v_priority=None  v=0 V  v_nominal_specify=off  v_nominal_unit=V  v_nominal_value=1  i_L_specify=on  i_L_priority=High  i_L=0 A  i_L_nominal_specify=off  i_L_nominal_unit=A  i_L_nominal_value=1
  LB_filt : fl_lib/Electrical/Electrical Elements/Inductor  l=6.2 mH  r=2 Ohm  g=1e-6 1/Ohm  i_specify=off  i_priority=None  i=0 A  i_nominal_specify=off  i_nominal_unit=A  i_nominal_value=1  v_specify=off  v_priority=None  v=0 V  v_nominal_specify=off  v_nominal_unit=V  v_nominal_value=1  i_L_specify=on  i_L_priority=High  i_L=0 A  i_L_nominal_specify=off  i_L_nominal_unit=A  i_L_nominal_value=1
  LC_filt : fl_lib/Electrical/Electrical Elements/Inductor  l=6.2 mH  r=2 Ohm  g=1e-6 1/Ohm  i_specify=off  i_priority=None  i=0 A  i_nominal_specify=off  i_nominal_unit=A  i_nominal_value=1  v_specify=off  v_priority=None  v=0 V  v_nominal_specify=off  v_nominal_unit=V  v_nominal_value=1  i_L_specify=on  i_L_priority=High  i_L=0 A  i_L_nominal_specify=off  i_L_nominal_unit=A  i_L_nominal_value=1
  Conn1 : PMIOPort  Port=1  Side=Left
  Conn2 : PMIOPort  Port=2  Side=Right
  Conn3 : PMIOPort  Port=3  Side=Left
  Conn4 : PMIOPort  Port=4  Side=Right
  Conn5 : PMIOPort  Port=5  Side=Left
  Conn6 : PMIOPort  Port=6  Side=Right
  connections:
  CdcS1/RConn1 -- Conn2/RConn1 -- LA_filt/RConn1
  CdcS2/LConn1 -- CdcS1/LConn1 -- CdcS3/LConn1
  CdcS3/RConn1 -- Conn4/RConn1 -- LB_filt/RConn1
  CdcS2/RConn1 -- Conn6/RConn1 -- LC_filt/RConn1
  LC_filt/LConn1 -- Conn5/RConn1
  LA_filt/LConn1 -- Conn1/RConn1
  LB_filt/LConn1 -- Conn3/RConn1

== system Back2BackSim1/inv1_(3legInverter)/Isens ==
  Current Sensor : fl_lib/Electrical/Electrical Sensors/Current Sensor
  PS-Simulink Converter : nesl_utility/PS-Simulink Converter  PhysicalDomain=network_engine_domain  SubClassName=ps_output  LeftPortType=input  RightPortType=output  PseudoPeriodic=off  Frequencies=[]  Unit=1  AffineConversion=off
  + : PMIOPort  Port=1  Side=Left
  - : PMIOPort  Port=2  Side=Right
  i : Outport
  wires:
  PS-Simulink Converter/1 -> i/1
  connections:
  PS-Simulink Converter/LConn1 -- Current Sensor/RConn1
  Current Sensor/RConn2 -- -/RConn1
  Current Sensor/LConn1 -- +/RConn1

== system Back2BackSim1/inv1_(3legInverter)/Isens1 ==
  Current Sensor : fl_lib/Electrical/Electrical Sensors/Current Sensor
  PS-Simulink Converter : nesl_utility/PS-Simulink Converter  PhysicalDomain=network_engine_domain  SubClassName=ps_output  LeftPortType=input  RightPortType=output  PseudoPeriodic=off  Frequencies=[]  Unit=1  AffineConversion=off
  + : PMIOPort  Port=1  Side=Left
  - : PMIOPort  Port=2  Side=Right
  i : Outport
  wires:
  PS-Simulink Converter/1 -> i/1
  connections:
  Current Sensor/LConn1 -- +/RConn1
  Current Sensor/RConn2 -- -/RConn1
  PS-Simulink Converter/LConn1 -- Current Sensor/RConn1

== system Back2BackSim1/inv1_(3legInverter)/Isens2 ==
  Current Sensor : fl_lib/Electrical/Electrical Sensors/Current Sensor
  PS-Simulink Converter : nesl_utility/PS-Simulink Converter  PhysicalDomain=network_engine_domain  SubClassName=ps_output  LeftPortType=input  RightPortType=output  PseudoPeriodic=off  Frequencies=[]  Unit=1  AffineConversion=off
  + : PMIOPort  Port=1  Side=Left
  - : PMIOPort  Port=2  Side=Right
  i : Outport
  wires:
  PS-Simulink Converter/1 -> i/1
  connections:
  PS-Simulink Converter/LConn1 -- Current Sensor/RConn1
  Current Sensor/RConn2 -- -/RConn1
  Current Sensor/LConn1 -- +/RConn1

== system Back2BackSim1/inv1_(3legInverter)/Steper1 ==
  In1 : Inport
  Product : Product
  Step : Step  Time=st_time3  SampleTime=0
  Out1 : Outport
  wires:
  Step/1 -> Product/2
  In1/1 -> Product/1
  Product/1 -> Out1/1

== system Back2BackSim1/inv1_(3legInverter)/Steper2 ==
  In1 : Inport
  Product : Product
  Step : Step  Time=st_time3  SampleTime=0
  Out1 : Outport
  wires:
  Product/1 -> Out1/1
  In1/1 -> Product/1
  Step/1 -> Product/2

== system Back2BackSim1/inv1_(3legInverter)/Steper3 ==
  In1 : Inport
  Product : Product
  Step : Step  Time=st_time3  SampleTime=0
  Out1 : Outport
  wires:
  Product/1 -> Out1/1
  In1/1 -> Product/1
  Step/1 -> Product/2

== system Back2BackSim1/inv1_(3legInverter)/Steper4 ==
  In1 : Inport
  Product : Product
  Step : Step  Time=st_time3  SampleTime=0
  Out1 : Outport
  wires:
  Step/1 -> Product/2
  In1/1 -> Product/1
  Product/1 -> Out1/1

== system Back2BackSim1/inv1_(3legInverter)/Steper5 ==
  In1 : Inport
  Product : Product
  Step : Step  Time=st_time3  SampleTime=0
  Out1 : Outport
  wires:
  Product/1 -> Out1/1
  In1/1 -> Product/1
  Step/1 -> Product/2

== system Back2BackSim1/inv1_(3legInverter)/Steper6 ==
  In1 : Inport
  Product : Product
  Step : Step  Time=st_time3  SampleTime=0
  Out1 : Outport
  wires:
  Step/1 -> Product/2
  In1/1 -> Product/1
  Product/1 -> Out1/1

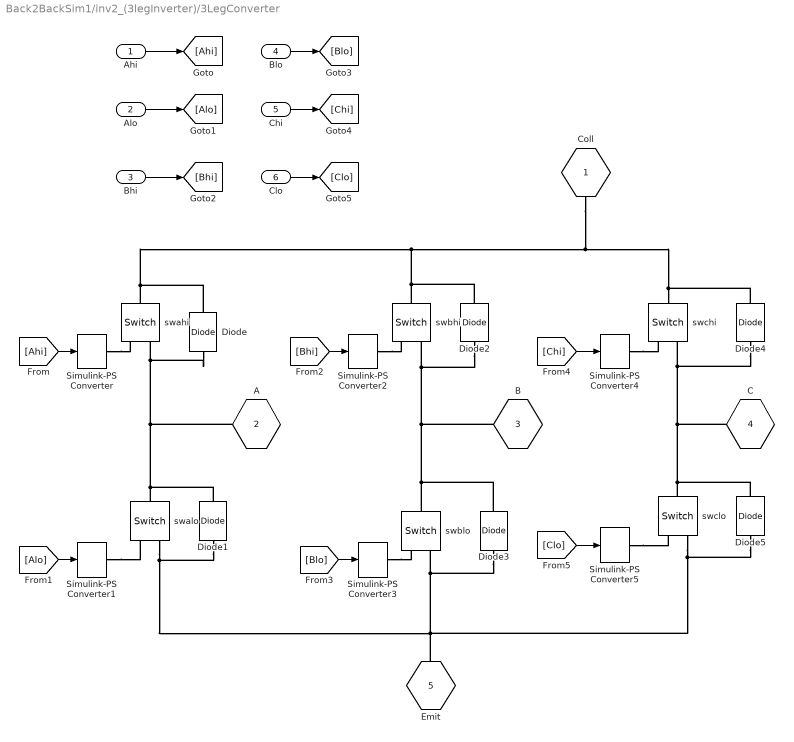
== system Back2BackSim1/inv2_(3legInverter)/3LegConverter ==
  Ahi : Inport
  Alo : Inport  Port=2
  Bhi : Inport  Port=3
  Blo : Inport  Port=4
  Chi : Inport  Port=5
  Clo : Inport  Port=6
  Diode{,1..5} (6 alike) : fl_lib/Electrical/Electrical Elements/Diode  Vf=0.6 V  Ron=0.3 Ohm  Goff=1e-8 1/Ohm  i_specify=off  i_priority=None  i=0 A  i_nominal_specify=off  i_nominal_unit=A  i_nominal_value=1  v_specify=off  v_priority=None  v=0 V  v_nominal_specify=off  v_nominal_unit=V  v_nominal_value=1
  Simulink-PS Converter{,1..5} (6 alike) : nesl_utility/Simulink-PS Converter  PhysicalDomain=network_engine_domain  SubClassName=ps_input  LeftPortType=input  RightPortType=output  PseudoPeriodic=off  Frequencies=[]  NoiseDistribution=none  NoiseParameters=[]  Unit=1  AffineConversion=off  FilteringAndDerivatives=zero  SimscapeFilterOrder=1  InputFilterTimeConstant=0.001  UdotUserProvided=1
  swahi : fl_lib/Electrical/Electrical Elements/Switch  R_closed=0.01 Ohm  G_open=1e-8 1/Ohm  Threshold=2  i_specify=off  i_priority=None  i=0 A  i_nominal_specify=off  i_nominal_unit=A  i_nominal_value=1  v_specify=off  v_priority=None  v=0 V  v_nominal_specify=off  v_nominal_unit=V  v_nominal_value=1
      settings: SourceProductName=Simscape
  swalo : fl_lib/Electrical/Electrical Elements/Switch  R_closed=0.01 Ohm  G_open=1e-8 1/Ohm  Threshold=2  i_specify=off  i_priority=None  i=0 A  i_nominal_specify=off  i_nominal_unit=A  i_nominal_value=1  v_specify=off  v_priority=None  v=0 V  v_nominal_specify=off  v_nominal_unit=V  v_nominal_value=1
      settings: SourceProductName=Simscape
  swbhi : fl_lib/Electrical/Electrical Elements/Switch  R_closed=0.01 Ohm  G_open=1e-8 1/Ohm  Threshold=2  i_specify=off  i_priority=None  i=0 A  i_nominal_specify=off  i_nominal_unit=A  i_nominal_value=1  v_specify=off  v_priority=None  v=0 V  v_nominal_specify=off  v_nominal_unit=V  v_nominal_value=1
      settings: SourceProductName=Simscape
  swblo : fl_lib/Electrical/Electrical Elements/Switch  R_closed=0.01 Ohm  G_open=1e-8 1/Ohm  Threshold=2  i_specify=off  i_priority=None  i=0 A  i_nominal_specify=off  i_nominal_unit=A  i_nominal_value=1  v_specify=off  v_priority=None  v=0 V  v_nominal_specify=off  v_nominal_unit=V  v_nominal_value=1
      settings: SourceProductName=Simscape
  swchi : fl_lib/Electrical/Electrical Elements/Switch  R_closed=0.01 Ohm  G_open=1e-8 1/Ohm  Threshold=2  i_specify=off  i_priority=None  i=0 A  i_nominal_specify=off  i_nominal_unit=A  i_nominal_value=1  v_specify=off  v_priority=None  v=0 V  v_nominal_specify=off  v_nominal_unit=V  v_nominal_value=1
      settings: SourceProductName=Simscape
  swclo : fl_lib/Electrical/Electrical Elements/Switch  R_closed=0.01 Ohm  G_open=1e-8 1/Ohm  Threshold=2  i_specify=off  i_priority=None  i=0 A  i_nominal_specify=off  i_nominal_unit=A  i_nominal_value=1  v_specify=off  v_priority=None  v=0 V  v_nominal_specify=off  v_nominal_unit=V  v_nominal_value=1
      settings: SourceProductName=Simscape
  Coll : PMIOPort  Port=1  Side=Right
  A : PMIOPort  Port=2  Side=Right
  B : PMIOPort  Port=3  Side=Right
  C : PMIOPort  Port=4  Side=Right
  Emit : PMIOPort  Port=5  Side=Right
  wires:
  Chi/1 -> [Chi]
  Blo/1 -> [Blo]
  [Chi] -> Simulink-PS Converter4/1
  Ahi/1 -> [Ahi]
  [Bhi] -> Simulink-PS Converter2/1
  Bhi/1 -> [Bhi]
  [Clo] -> Simulink-PS Converter5/1
  [Blo] -> Simulink-PS Converter3/1
  Alo/1 -> [Alo]
  Clo/1 -> [Clo]
  [Ahi] -> Simulink-PS Converter/1
  [Alo] -> Simulink-PS Converter1/1
  connections:
  swchi/RConn2 -- Diode4/LConn1 -- C/RConn1 -- Diode5/RConn1 -- swclo/LConn1
  swchi/LConn1 -- Diode4/RConn1 -- Coll/RConn1 -- swbhi/LConn1 -- Diode2/RConn1 -- Diode/RConn1 -- swahi/LConn1
  Diode1/RConn1 -- swahi/RConn2 -- Diode/LConn1 -- A/RConn1 -- swalo/LConn1
  Simulink-PS Converter1/RConn1 -- swalo/RConn1
  Simulink-PS Converter2/RConn1 -- swbhi/RConn1
  Simulink-PS Converter3/RConn1 -- swblo/RConn1
  swbhi/RConn2 -- Diode2/LConn1 -- B/RConn1 -- Diode3/RConn1 -- swblo/LConn1
  Simulink-PS Converter/RConn1 -- swahi/RConn1
  Simulink-PS Converter5/RConn1 -- swclo/RConn1
  Simulink-PS Converter4/RConn1 -- swchi/RConn1
  Diode1/LConn1 -- swclo/RConn2 -- Diode5/LConn1 -- Emit/RConn1 -- swblo/RConn2 -- Diode3/LConn1 -- swalo/RConn2

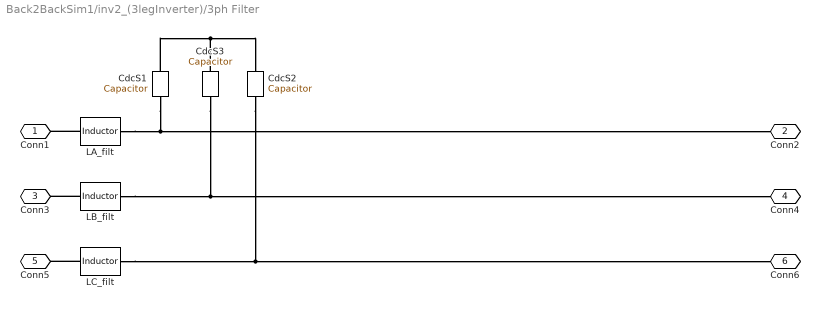
== system Back2BackSim1/inv2_(3legInverter)/3ph Filter ==
  CdcS1 : fl_lib/Electrical/Electrical Elements/Capacitor  c=3.5 uF  r=1e-6 Ohm  g=0 1/Ohm  i_specify=off  i_priority=None  i=0 A  i_nominal_specify=off  i_nominal_unit=A  i_nominal_value=1  v_specify=off  v_priority=None  v=0 V  v_nominal_specify=off  v_nominal_unit=V  v_nominal_value=1  vc_specify=on  vc_priority=High  vc=0 V  vc_nominal_specify=off  vc_nominal_unit=V  vc_nominal_value=1
  CdcS2 : fl_lib/Electrical/Electrical Elements/Capacitor  c=3.5 uF  r=1e-6 Ohm  g=0 1/Ohm  i_specify=off  i_priority=None  i=0 A  i_nominal_specify=off  i_nominal_unit=A  i_nominal_value=1  v_specify=off  v_priority=None  v=0 V  v_nominal_specify=off  v_nominal_unit=V  v_nominal_value=1  vc_specify=on  vc_priority=High  vc=0 V  vc_nominal_specify=off  vc_nominal_unit=V  vc_nominal_value=1
  CdcS3 : fl_lib/Electrical/Electrical Elements/Capacitor  c=3.5 uF  r=1e-6 Ohm  g=0 1/Ohm  i_specify=off  i_priority=None  i=0 A  i_nominal_specify=off  i_nominal_unit=A  i_nominal_value=1  v_specify=off  v_priority=None  v=0 V  v_nominal_specify=off  v_nominal_unit=V  v_nominal_value=1  vc_specify=on  vc_priority=High  vc=0 V  vc_nominal_specify=off  vc_nominal_unit=V  vc_nominal_value=1
  LA_filt : fl_lib/Electrical/Electrical Elements/Inductor  l=6.2 mH  r=0.1 Ohm  g=1e-6 1/Ohm  i_specify=off  i_priority=None  i=0 A  i_nominal_specify=off  i_nominal_unit=A  i_nominal_value=1  v_specify=off  v_priority=None  v=0 V  v_nominal_specify=off  v_nominal_unit=V  v_nominal_value=1  i_L_specify=on  i_L_priority=High  i_L=0 A  i_L_nominal_specify=off  i_L_nominal_unit=A  i_L_nominal_value=1
  LB_filt : fl_lib/Electrical/Electrical Elements/Inductor  l=6.2 mH  r=2 Ohm  g=1e-6 1/Ohm  i_specify=off  i_priority=None  i=0 A  i_nominal_specify=off  i_nominal_unit=A  i_nominal_value=1  v_specify=off  v_priority=None  v=0 V  v_nominal_specify=off  v_nominal_unit=V  v_nominal_value=1  i_L_specify=on  i_L_priority=High  i_L=0 A  i_L_nominal_specify=off  i_L_nominal_unit=A  i_L_nominal_value=1
  LC_filt : fl_lib/Electrical/Electrical Elements/Inductor  l=6.2 mH  r=2 Ohm  g=1e-6 1/Ohm  i_specify=off  i_priority=None  i=0 A  i_nominal_specify=off  i_nominal_unit=A  i_nominal_value=1  v_specify=off  v_priority=None  v=0 V  v_nominal_specify=off  v_nominal_unit=V  v_nominal_value=1  i_L_specify=on  i_L_priority=High  i_L=0 A  i_L_nominal_specify=off  i_L_nominal_unit=A  i_L_nominal_value=1
  Conn1 : PMIOPort  Port=1  Side=Left
  Conn2 : PMIOPort  Port=2  Side=Right
  Conn3 : PMIOPort  Port=3  Side=Left
  Conn4 : PMIOPort  Port=4  Side=Right
  Conn5 : PMIOPort  Port=5  Side=Left
  Conn6 : PMIOPort  Port=6  Side=Right
  connections:
  LB_filt/LConn1 -- Conn3/RConn1
  LA_filt/LConn1 -- Conn1/RConn1
  LC_filt/LConn1 -- Conn5/RConn1
  LC_filt/RConn1 -- Conn6/RConn1 -- CdcS2/RConn1
  LB_filt/RConn1 -- Conn4/RConn1 -- CdcS3/RConn1
  CdcS3/LConn1 -- CdcS1/LConn1 -- CdcS2/LConn1
  LA_filt/RConn1 -- Conn2/RConn1 -- CdcS1/RConn1

== system Back2BackSim1/inv2_(3legInverter)/Isens ==
  Current Sensor : fl_lib/Electrical/Electrical Sensors/Current Sensor
  PS-Simulink Converter : nesl_utility/PS-Simulink Converter  PhysicalDomain=network_engine_domain  SubClassName=ps_output  LeftPortType=input  RightPortType=output  PseudoPeriodic=off  Frequencies=[]  Unit=1  AffineConversion=off
  + : PMIOPort  Port=1  Side=Left
  - : PMIOPort  Port=2  Side=Right
  i : Outport
  wires:
  PS-Simulink Converter/1 -> i/1
  connections:
  Current Sensor/LConn1 -- +/RConn1
  Current Sensor/RConn2 -- -/RConn1
  PS-Simulink Converter/LConn1 -- Current Sensor/RConn1

== system Back2BackSim1/inv2_(3legInverter)/Isens1 ==
  Current Sensor : fl_lib/Electrical/Electrical Sensors/Current Sensor
  PS-Simulink Converter : nesl_utility/PS-Simulink Converter  PhysicalDomain=network_engine_domain  SubClassName=ps_output  LeftPortType=input  RightPortType=output  PseudoPeriodic=off  Frequencies=[]  Unit=1  AffineConversion=off
  + : PMIOPort  Port=1  Side=Left
  - : PMIOPort  Port=2  Side=Right
  i : Outport
  wires:
  PS-Simulink Converter/1 -> i/1
  connections:
  PS-Simulink Converter/LConn1 -- Current Sensor/RConn1
  Current Sensor/RConn2 -- -/RConn1
  Current Sensor/LConn1 -- +/RConn1

== system Back2BackSim1/inv2_(3legInverter)/Isens2 ==
  Current Sensor : fl_lib/Electrical/Electrical Sensors/Current Sensor
  PS-Simulink Converter : nesl_utility/PS-Simulink Converter  PhysicalDomain=network_engine_domain  SubClassName=ps_output  LeftPortType=input  RightPortType=output  PseudoPeriodic=off  Frequencies=[]  Unit=1  AffineConversion=off
  + : PMIOPort  Port=1  Side=Left
  - : PMIOPort  Port=2  Side=Right
  i : Outport
  wires:
  PS-Simulink Converter/1 -> i/1
  connections:
  Current Sensor/LConn1 -- +/RConn1
  Current Sensor/RConn2 -- -/RConn1
  PS-Simulink Converter/LConn1 -- Current Sensor/RConn1

== system Back2BackSim1/inv2_(3legInverter)/Steper1 ==
  In1 : Inport
  Product : Product
  Step : Step  Time=st_time3  SampleTime=0
  Out1 : Outport
  wires:
  Product/1 -> Out1/1
  In1/1 -> Product/1
  Step/1 -> Product/2

== system Back2BackSim1/inv2_(3legInverter)/Steper2 ==
  In1 : Inport
  Product : Product
  Step : Step  Time=st_time3  SampleTime=0
  Out1 : Outport
  wires:
  Step/1 -> Product/2
  In1/1 -> Product/1
  Product/1 -> Out1/1

== system Back2BackSim1/inv2_(3legInverter)/Steper3 ==
  In1 : Inport
  Product : Product
  Step : Step  Time=st_time3  SampleTime=0
  Out1 : Outport
  wires:
  Step/1 -> Product/2
  In1/1 -> Product/1
  Product/1 -> Out1/1

== system Back2BackSim1/inv2_(3legInverter)/Steper4 ==
  In1 : Inport
  Product : Product
  Step : Step  Time=st_time3  SampleTime=0
  Out1 : Outport
  wires:
  Product/1 -> Out1/1
  In1/1 -> Product/1
  Step/1 -> Product/2

== system Back2BackSim1/inv2_(3legInverter)/Steper5 ==
  In1 : Inport
  Product : Product
  Step : Step  Time=st_time3  SampleTime=0
  Out1 : Outport
  wires:
  Step/1 -> Product/2
  In1/1 -> Product/1
  Product/1 -> Out1/1

== system Back2BackSim1/inv2_(3legInverter)/Steper6 ==
  In1 : Inport
  Product : Product
  Step : Step  Time=st_time3  SampleTime=0
  Out1 : Outport
  wires:
  Product/1 -> Out1/1
  In1/1 -> Product/1
  Step/1 -> Product/2

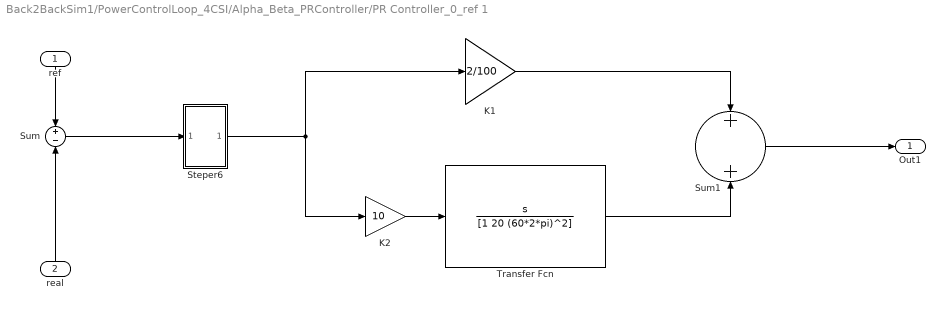
== system Back2BackSim1/PowerControlLoop_4CSI/Alpha_Beta_PRController/PR Controller_0_ref 1 ==
  ref : Inport
  real : Inport  Port=2
  K1 : Gain  Gain=2/100
  K2 : Gain  Gain=10
  Steper6 : Subsystem
  Sum : Sum  Inputs=+-
  Sum1 : Sum  Inputs=+|+
  Transfer Fcn : TransferFcn  Numerator=[1 0]  Denominator=[1 20 (60*2*pi)^2]
  Out1 : Outport
  wires:
  Sum1/1 -> Out1/1
  Steper6/1(Out1) -> K2/1, K1/1
  K2/1 -> Transfer Fcn/1
  Transfer Fcn/1 -> Sum1/2
  K1/1 -> Sum1/1
  Sum/1 -> Steper6/1(In1)
  ref/1 -> Sum/1
  real/1 -> Sum/2

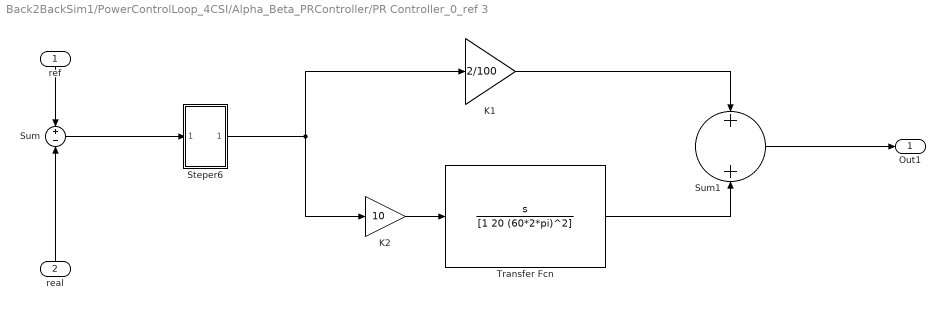
== system Back2BackSim1/PowerControlLoop_4CSI/Alpha_Beta_PRController/PR Controller_0_ref 3 ==
  ref : Inport
  real : Inport  Port=2
  K1 : Gain  Gain=2/100
  K2 : Gain  Gain=10
  Steper6 : Subsystem
  Sum : Sum  Inputs=+-
  Sum1 : Sum  Inputs=+|+
  Transfer Fcn : TransferFcn  Numerator=[1 0]  Denominator=[1 20 (60*2*pi)^2]
  Out1 : Outport
  wires:
  real/1 -> Sum/2
  ref/1 -> Sum/1
  Sum/1 -> Steper6/1(In1)
  K1/1 -> Sum1/1
  Transfer Fcn/1 -> Sum1/2
  K2/1 -> Transfer Fcn/1
  Steper6/1(Out1) -> K1/1, K2/1
  Sum1/1 -> Out1/1

== system Back2BackSim1/PowerControlLoop_4CSI/Alpha_Beta_PRController/PR Controller_0_ref 1/Steper6 ==
  In1 : Inport
  Product : Product
  Step : Step  Time=st_time3  SampleTime=0
  Out1 : Outport
  wires:
  Step/1 -> Product/2
  In1/1 -> Product/1
  Product/1 -> Out1/1

== system Back2BackSim1/PowerControlLoop_4CSI/Alpha_Beta_PRController/PR Controller_0_ref 3/Steper6 ==
  In1 : Inport
  Product : Product
  Step : Step  Time=st_time3  SampleTime=0
  Out1 : Outport
  wires:
  Product/1 -> Out1/1
  In1/1 -> Product/1
  Step/1 -> Product/2

== matlab function Back2BackSim1/inv1_(3legInverter)/not_pwm1 ==
  data: u input; y output
function y = fcn(u)
%#codegen

if(u==0 || u<0)
    a=5;
else
    a=0;
end;

y = a;

== matlab function Back2BackSim1/inv1_(3legInverter)/not_pwm ==
  data: u input; y output
function y = fcn(u)
%#codegen

if(u==0 || u<0)
    a=15;
else
    a=0;
end;

y = a;

== matlab function Back2BackSim1/inv1_(3legInverter)/not_pwm2 ==
  data: u input; y output
function y = fcn(u)
%#codegen

if(u==0 || u<0)
    a=5;
else
    a=0;
end;

y = a;

== matlab function Back2BackSim1/inv2_(3legInverter)/not_pwm ==
  data: u input; y output
function y = fcn(u)
%#codegen

if(u==0 || u<0)
    a=15;
else
    a=0;
end;

y = a;

== matlab function Back2BackSim1/inv2_(3legInverter)/not_pwm1 ==
  data: u input; y output
function y = fcn(u)
%#codegen

if(u==0 || u<0)
    a=5;
else
    a=0;
end;

y = a;

== matlab function Back2BackSim1/inv2_(3legInverter)/not_pwm2 ==
  data: u input; y output
function y = fcn(u)
%#codegen

if(u==0 || u<0)
    a=5;
else
    a=0;
end;

y = a;
